simulink library "TSAA_Altitude_Error"  (R2016b)
settings: Solver=VariableStepAuto  StartTime=0.0  StopTime=10.0  RelTol=1e-3
undefined symbols (not defined in the file or in its folder): altQuant_ft, randomSeed
undefined symbols (not defined in the file): lambdaRandomSeed
settings Model: Creator=RA24876  LastModifiedBy=RA24876

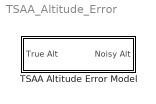
== system TSAA_Altitude_Error ==
  TSAA Altitude Error Model : Subsystem  mask{ac_id=1, perfect=false, lambdaSeed=lambdaRandomSeed, randomSeed=randomSeed, altQuant_ft=altQuant_ft, dt_s=0}
      mask prompts: ac_id "Aircraft ID (ownship=1)"; perfect "Use Perfect Altimetry"; lambdaSeed "Lambda Random Seed"; randomSeed "Random Seed"; altQuant_ft "Altitude Quantization (ft)"; dt_s "Sample Time"

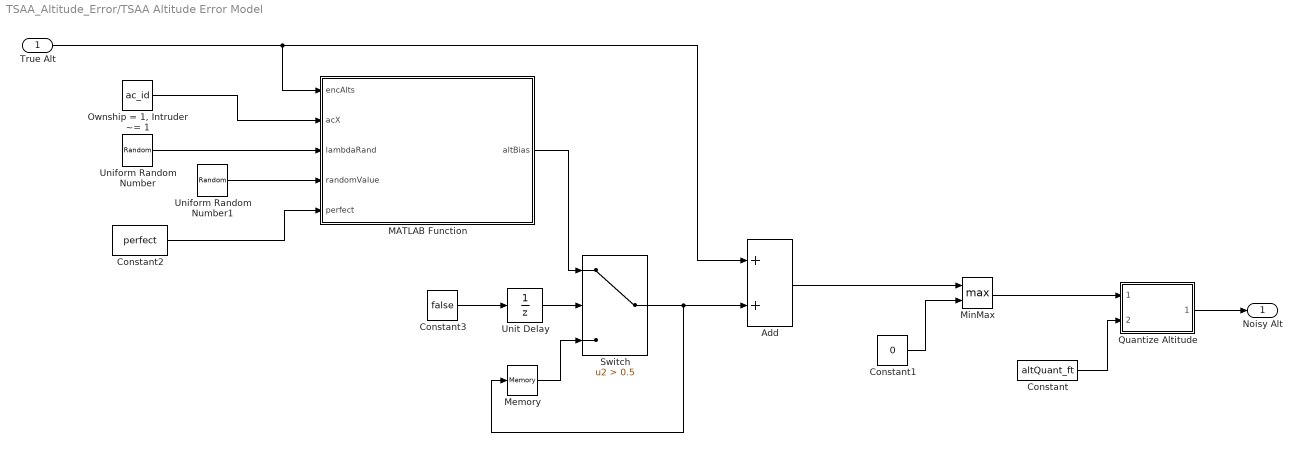
== system TSAA_Altitude_Error/TSAA Altitude Error Model ==
  True Alt : Inport
  Add : Sum
  Constant : Constant  Value=altQuant_ft
  Constant1 : Constant  Value=0
  Constant2 : Constant  Value=perfect
  Constant3 : Constant  Value=false
  MATLAB Function : MATLAB Function  TreatAsAtomicUnit=on
  Memory : Memory
  MinMax : MinMax  Function=max  Inputs=2
  "Ownship = 1, Intruder ~= 1" : Constant  Value=ac_id
  Quantize Altitude : Subsystem
  Switch : Switch  Criteria=u2 > Threshold  Threshold=0.5
  Uniform Random Number : UniformRandomNumber  Minimum=0  Seed=lambdaSeed  SampleTime=dt_s
  Uniform Random Number1 : UniformRandomNumber  Minimum=0  Seed=randomSeed  SampleTime=dt_s
  Unit Delay : UnitDelay  InitialCondition=true  SampleTime=-1
  Noisy Alt : Outport
  wires:
  Constant/1 -> Quantize Altitude/2(Quant_level)
  Add/1 -> MinMax/1
  Memory/1 -> Switch/3
  Switch/1 -> Memory/1, Add/2
  Unit Delay/1 -> Switch/2
  Constant3/1 -> Unit Delay/1
  MATLAB Function/1(altBias) -> Switch/1
  Uniform Random Number1/1 -> MATLAB Function/4(randomValue)
  Uniform Random Number/1 -> MATLAB Function/3(lambdaRand)
  True Alt/1 -> MATLAB Function/1(encAlts), Add/1
  "Ownship = 1, Intruder ~= 1"/1 -> MATLAB Function/2(acX)
  Constant1/1 -> MinMax/2
  MinMax/1 -> Quantize Altitude/1(Altitude)
  Quantize Altitude/1(Quantized Alt) -> Noisy Alt/1
  Constant2/1 -> MATLAB Function/5(perfect)

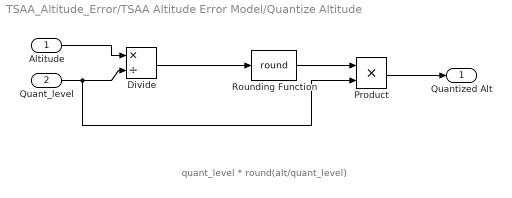
== system TSAA_Altitude_Error/TSAA Altitude Error Model/Quantize Altitude ==
  note: quant_level * round(alt/quant_level)
  Altitude : Inport
  Quant_level : Inport  Port=2
  Divide : Product  Inputs=*/
  Product : Product
  Rounding Function : Rounding  Operator=round
  Quantized Alt : Outport
  wires:
  Product/1 -> Quantized Alt/1
  Rounding Function/1 -> Product/1
  Divide/1 -> Rounding Function/1
  Quant_level/1 -> Divide/2, Product/2
  Altitude/1 -> Divide/1

== matlab function TSAA_Altitude_Error/TSAA Altitude Error Model/MATLAB Function ==
  data: encAlts input; altBias output; acX input; lambdaRand input; randomValue input; perfect input
function altBias  = degradeAlt(encAlts, acX, lambdaRand, randomValue, perfect)

altBias = TSAA_Model_External_Functions.degradeAlt(encAlts, acX, lambdaRand, randomValue, perfect);
